simulink model "crane_model_v02_sim_improved"  (R2021a)
settings: Solver=ode23t  StartTime=0.0  StopTime=120.0  RelTol=1e-3
model workspace (MAT data in the model file):
  I_xx_0 : Simulink.Parameter (value not decoded)
  I_xx_1 : Simulink.Parameter (value not decoded)
  I_xx_2 : Simulink.Parameter (value not decoded)
  I_xx_b : Simulink.Parameter (value not decoded)
  I_xx_b1 : Simulink.Parameter (value not decoded)
  I_xx_b2 : Simulink.Parameter (value not decoded)
  I_xx_c1 : Simulink.Parameter (value not decoded)
  I_xx_c2 : Simulink.Parameter (value not decoded)
  I_yy_0 : Simulink.Parameter (value not decoded)
  I_yy_1 : Simulink.Parameter (value not decoded)
  I_yy_2 : Simulink.Parameter (value not decoded)
  I_yy_b : Simulink.Parameter (value not decoded)
  I_yy_b1 : Simulink.Parameter (value not decoded)
  I_yy_b2 : Simulink.Parameter (value not decoded)
  I_yy_c1 : Simulink.Parameter (value not decoded)
  I_yy_c2 : Simulink.Parameter (value not decoded)
  I_zz_0 : Simulink.Parameter (value not decoded)
  I_zz_1 : Simulink.Parameter (value not decoded)
  I_zz_2 : Simulink.Parameter (value not decoded)
  I_zz_b : Simulink.Parameter (value not decoded)
  I_zz_b1 : Simulink.Parameter (value not decoded)
  I_zz_b2 : Simulink.Parameter (value not decoded)
  I_zz_c1 : Simulink.Parameter (value not decoded)
  I_zz_c2 : Simulink.Parameter (value not decoded)
  J_a : Simulink.Parameter (value not decoded)
  Sig : Simulink.Signal (value not decoded)
  Sig1 : Simulink.Signal (value not decoded)
  a1_l : Simulink.Parameter (value not decoded)
  a1_t : Simulink.Parameter (value not decoded)
  a2_l : Simulink.Parameter (value not decoded)
  a2_t : Simulink.Parameter (value not decoded)
  arm_d : Simulink.Parameter (value not decoded)
  arm_w : Simulink.Parameter (value not decoded)
  b_1 : Simulink.Parameter (value not decoded)
  b_2 : Simulink.Parameter (value not decoded)
  h_base : Simulink.Parameter (value not decoded)
  l_0 : Simulink.Parameter (value not decoded)
  l_1 : Simulink.Parameter (value not decoded)
  l_2 : Simulink.Parameter (value not decoded)
  l_a1_rod : Simulink.Parameter (value not decoded)
  l_a2_rod : Simulink.Parameter (value not decoded)
  l_b1x : Simulink.Parameter (value not decoded)
  l_b1z : Simulink.Parameter (value not decoded)
  l_b2 : Simulink.Parameter (value not decoded)
  l_b4x : Simulink.Parameter (value not decoded)
  l_b4y : Simulink.Parameter (value not decoded)
  l_c1x : Simulink.Parameter (value not decoded)
  l_c1y : Simulink.Parameter (value not decoded)
  l_c2 : Simulink.Parameter (value not decoded)
  l_c3x : Simulink.Parameter (value not decoded)
  l_c3y : Simulink.Parameter (value not decoded)
  l_set = 0.5
  m_0 : Simulink.Parameter (value not decoded)
  m_1 : Simulink.Parameter (value not decoded)
  m_2 : Simulink.Parameter (value not decoded)
  m_b1 : Simulink.Parameter (value not decoded)
  m_b2 : Simulink.Parameter (value not decoded)
  m_base : Simulink.Parameter (value not decoded)
  m_c1 : Simulink.Parameter (value not decoded)
  m_c2 : Simulink.Parameter (value not decoded)
  m_p : Simulink.Parameter (value not decoded)
  r_base : Simulink.Parameter (value not decoded)
  r_cyl : Simulink.Parameter (value not decoded)
  r_cyl_0 : Simulink.Parameter (value not decoded)
  x_set = 3.7
  y_set = 0.3
  z_set = 2.2
symbols that are objects in the model workspace (value not decoded): a1_l, a1_t, a2_l, a2_t, arm_d, arm_w, h_base, I_xx_0, I_xx_1, I_xx_2, I_xx_b, I_xx_b1, I_xx_b2, I_xx_c1, I_xx_c2, I_yy_0, I_yy_1, I_yy_2, I_yy_b, I_yy_b1, I_yy_b2, I_yy_c1, I_yy_c2, I_zz_0, I_zz_1, I_zz_2, I_zz_b, I_zz_b1, I_zz_b2, I_zz_c1, I_zz_c2, l_0, l_1, l_2, l_a1_rod, l_a2_rod, l_b1x, l_b1z, l_b2, l_b4x, l_b4y, l_c1x, l_c1y, l_c2, l_c3x, l_c3y, m_0, m_1, m_2, m_b1, m_b2, m_base, m_c1, m_c2
undefined symbols (not defined in the file): sigbuilder_block, X, Y, Z
libraries: sm_lib x103, nesl_utility x23, pid_lib x7, fuzblock x1
(part 5 of 5)

== matlab function crane_model_v02_sim_improved/Sway Modifier/Inverse Kinematics ==
  data: u input; theta_0 output; d_1 output; d_2 output
function [theta_0, d_1, d_2] = crane_model_v02_ik(u)
    x_d = u(1); 
    y_d = u(2); 
    z_d = u(3); 
    l_0 = 2.1; 
    l_1 = 2.3; 
    l_2 = 2.1; 

    l_b1x = 0.3; 
    l_b1z = 0.2; 
    l_b4x = 0.5; 
    l_b4y = 0.15; 
    l_c1x = 1.1; 
    l_c1y = 0.15; 
    l_c3x = 0.65; 
    l_c3y = 0.15; 
    l_b2 = 1.0; 
    l_c2 = 0.6; 

    a_1 = sqrt(l_b4x^2+l_b4y^2); 
    b_1 = sqrt(l_b1x^2+(l_0-l_b1x)^2); 
    a_2 = sqrt(l_c1x^2+l_c1y^2); 
    b_2 = sqrt(l_c3x^2+l_c3y^2); 
    
    theta_0 = atan2(y_d, x_d); 

    gamma = l_2^2 - l_1^2 - (l_0 - z_d)^2 ...
        - (x_d*cos(theta_0)+y_d*sin(theta_0))^2; 

    rho = 2*l_1*sqrt((x_d*cos(theta_0)+y_d*sin(theta_0))^2 + (l_0-z_d)^2); 

    t1p = atan((x_d*cos(theta_0)+y_d*sin(theta_0)) / (l_0-z_d)); 

    theta_1 = atan((gamma/rho) / (-sqrt(1-(gamma/rho)^2)))-t1p; 

    theta_2 = atan((l_0 - l_1*sin(theta_1) - z_d) / ...
        (x_d*cos(theta_0) + y_d*sin(theta_0)-l_1*cos(theta_1))) - theta_1; 
    
    % fprintf('theta_2: %f\n', theta_2)

    d_1 = sqrt(a_1^2 + b_1^2 - 2*a_1*b_1*...
        cos(pi/2-theta_1-atan(l_b1x/(l_0-l_b1z))-atan(l_b4y/l_b4x))) - l_b2; 
    d_2 = sqrt(a_2^2 + b_2^2 - 2*a_2*b_2*...
        cos(pi - theta_2 - atan(l_c1y/l_c1x) - atan(l_c3y/l_c3x))) - l_c2; 
end

== matlab function crane_model_v02_sim_improved/Sway Modifier/Transform to R6 ==
  data: u input; x_6 output
function x_6  = fcn(u)
    t_0 = u(1); 
%     d_1 = u(2); 
%     d_2 = u(3); 
    t_1 = u(4); 
    t_2 = u(5); 
    x = u(6); 
    y = u(7); 
    z = u(8); 
    l = u(9); 
    t_3 = u(10); 
    t_4 = u(11); 
    x_e = x - sin(t_0)*sin(t_4)*l + cos(t_0)*cos(t_4)*cos(t_1+t_2+t_3)*l; 
    y_e = y - cos(t_0)*sin(t_4)*l + sin(t_0)*cos(t_4)*cos(t_1+t_2+t_3)*l;
    z_e = z - cos(t_4)*sin(t_1+t_2+t_3)*l; 
    l_e = l; 
    x_6 = [x_e, y_e, z_e, l_e]; 
    
end

== matlab function crane_model_v02_sim_improved/Sway Modifier/Transform to R3 ==
  data: u input; x_3 output
function x_3  = fcn(u)
    t_0 = u(1); 
    t_1 = u(2); 
    t_2 = u(3); 
    l = u(4); 
    x = u(5); 
    y = u(6); 
    z = u(7); 
%     l = u(8); 
    t_3 = u(9); 
    t_4 = u(10); 
    
    x_e = x + sin(t_0)*sin(t_4)*l - cos(t_0)*cos(t_4)*cos(t_1+t_2+t_3)*l; 
    y_e = y + cos(t_0)*sin(t_4)*l - sin(t_0)*cos(t_4)*cos(t_1+t_2+t_3)*l;
    z_e = z + cos(t_4)*sin(t_1+t_2+t_3)*l; 
    
    x_3 = [x_e, y_e, z_e]; 
end

== matlab function crane_model_v02_sim_improved/Sway Modifier/extract_t1t2 ==
  data: u input; t_1 output; t_2 output
function [t_1, t_2] = fcn(u)
    t_1 = u(4); 
    t_2 = u(5); 
y = u;

== matlab function crane_model_v02_sim_improved/To Bus/To Bus ==
  data: u input; t_0 output; d_1 output; d_2 output; l_3 output
function [t_0, d_1, d_2, l_3] = convert_to_struct(u)
t_0 = u(1); 
d_1 = u(2); 
d_2 = u(3); 
l_3 = u(6); 

end

== matlab function crane_model_v02_sim_improved/To Bus1/To Bus ==
  data: u input; x_dm output; y_dm output; z_dm output; l_dm output
function [x_dm, y_dm, z_dm, l_dm] = convert_to_struct(u)
x_dm = u(1); 
y_dm = u(2); 
z_dm = u(3); 
l_dm = u(4); 

end

== matlab function crane_model_v02_sim_improved/Controller/Tuner d_1 ==
  data: e_d1 input; k_p_d1 output; k_i_d1 output; k_d_d1 output; m input
function [k_p_d1, k_i_d1, k_d_d1] = fcn(e_d1, m)

if ~m
    m = 200; 
end

mul_f = 3; 
k_p = 3.0e6; 
k_i = 3.0e6; 
k_d = 3.0e6; 

k_p_d1 = k_p + mul_f*k_p * exp(-40*abs(e_d1)) + m*1000;
k_i_d1 = k_i + mul_f*k_i * exp(-40*abs(e_d1)); 
k_d_d1 = k_d + mul_f*k_d * exp(-40*abs(e_d1)); 
end
